simulink model "WholeSys0720_Simplified"  (Simulink 7.5)
settings: Solver=ode15s  StartTime=0.0  StopTime=10.0  MaxStep=0.2  RelTol=1e-3
undefined symbols (not defined in the file or in its folder): des_attributefunction_support, des_figposition, des_subsystemblock, des_subsysteminport, des_subsystemoutport, des_subsystemsupportblock, DiscIntNeverNeededParam, mm, Radius, sigbuilder_block, X, Y
libraries: simeventssink1 x10, simeventsattributes2 x5, simeventsgenerators1 x4, dspmathops x3, simeventstranslate1 x3, dspsigops x2, dspsrcs4 x2, simeventsgates1 x1, simeventsrouting1 x1, simeventsserver1 x1
settings Model: Creator=Administrator  LastModifiedBy=Administrator
settings DebuggingCC: StrictBusMsg=Warning
settings SimEventsCC: propDiagAttribOutput=1  propDiagFcnCallOutput=1  propDiagStatOutput=0

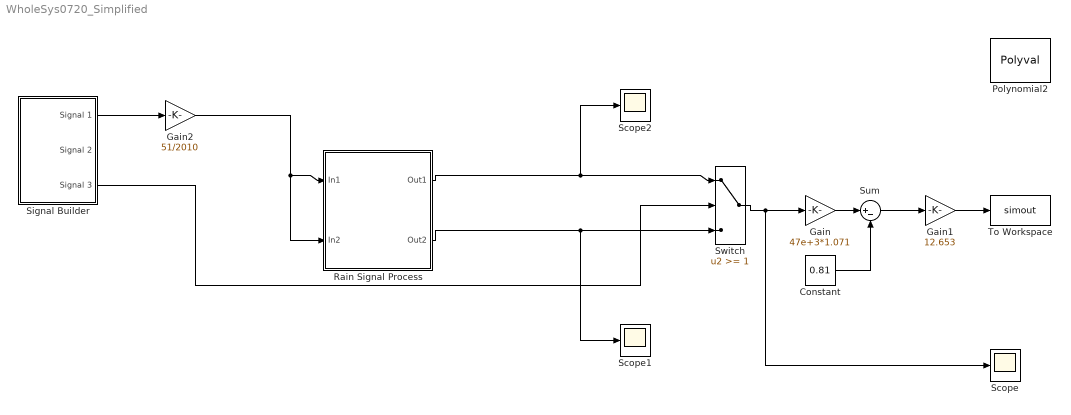
== system WholeSys0720_Simplified ==
  Constant : Constant  Value=0.81  OutDataType=sfix(16)  OutScaling=2^0
  Gain : Gain  Gain=47e+3*1.071  ParameterDataType=sfix(16)  ParameterScaling=2^0  OutDataType=sfix(16)  OutScaling=2^0
  Gain1 : Gain  Gain=12.653  ParameterDataType=sfix(16)  ParameterScaling=2^0  OutDataType=sfix(16)  OutScaling=2^0
  Gain2 : Gain  Gain=51/2010  ParameterDataType=fixdt(1, 16)  ParameterScaling=2^0  OutDataType=fixdt(1, 16)  OutScaling=2^0
  Polynomial2 : Polyval  Coefs=[ 1 ]
  Rain Signal Process : Subsystem
  Scope : Scope
      settings: YMin=-0.5  YMax=1.5  MaxDataPoints=100000
  Scope1 : Scope
      settings: YMin=-0.5  YMax=1  SaveName=ScopeData2  MaxDataPoints=100000
  Scope2 : Scope
      settings: YMin=-0.5  YMax=1  SaveName=ScopeData9  MaxDataPoints=100000
  Signal Builder : Subsystem  Tag=STV Subsys  LoadFcn=sigbuilder_block('load');  StartFcn=sigbuilder_block('start');  StopFcn=sigbuilder_block('stop');  ClipboardFcn=sigbuilder_block('clipboard');  mask(Sigbuilder block){}
      mask help: Create and generate interchangeable groups of signals whose waveforms are piecewise linear.
      mask init:
      | if ~strcmp(get_param(bdroot(gcbh),'SimulationStatus'),'stopped') tuvar = sigbuilder_block('maskInit'); end
      settings: CopyFcn=sigbuilder_block('copy');  DeleteFcn=sigbuilder_block('delete');  ModelCloseFcn=sigbuilder_block('modelClose');  PreSaveFcn=sigbuilder_block('preSave');  NameChangeFcn=sigbuilder_block('namechange');  OpenFcn=sigbuilder_block('open',[437.25 199.5 550.5 399.75 ]);  CloseFcn=sigbuilder_block('close');
      mask Display: plot(0,0,100,100,[10,10,40,40,10],[80,20,20,80,80],[40,10],[50,50], [40,27,10],[65,72,56],[40,25,25,10],[28,28,43,43]);
  Sum : Sum  Inputs=|+-  OutDataType=sfix(16)  OutScaling=2^0
  Switch : Switch  Threshold=1  OutDataType=fixdt(1, 16)  OutScaling=2^0
  To Workspace : ToWorkspace  VariableName=simout  SampleTime=-1  SaveFormat=Structure
  wires:
  Gain2/1 -> Rain Signal Process/1(In1), Rain Signal Process/2(In2)
  Gain/1 -> Sum/1
  Constant/1 -> Sum/2
  Sum/1 -> Gain1/1
  Gain1/1 -> To Workspace/1
  Rain Signal Process/1(Out1) -> Switch/1, Scope2/1
  Rain Signal Process/2(Out2) -> Switch/3, Scope1/1
  Switch/1 -> Gain/1, Scope/1
  Signal Builder/1(Signal 1) -> Gain2/1
  Signal Builder/3(Signal 3) -> Switch/2

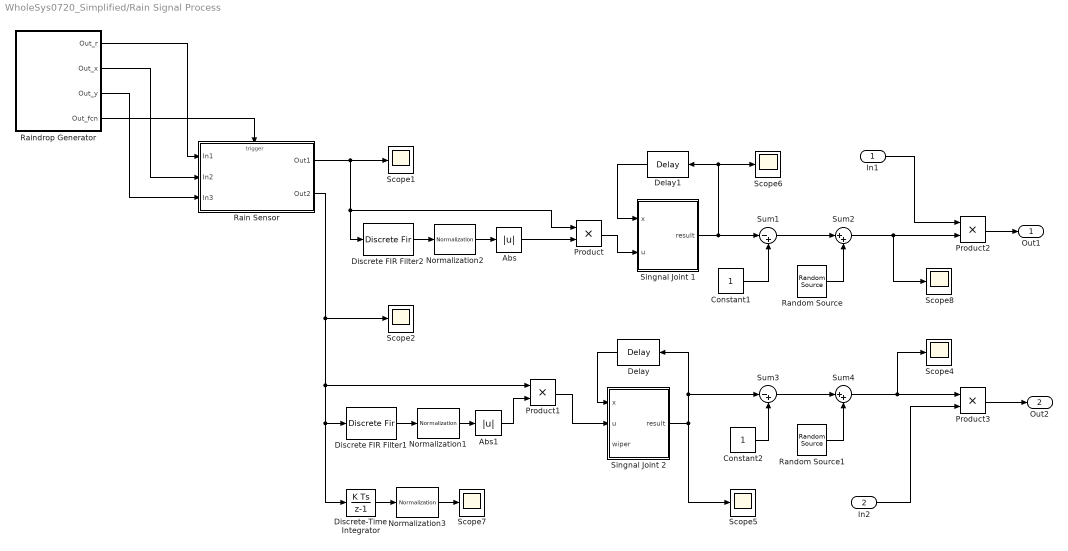
== system WholeSys0720_Simplified/Rain Signal Process ==
  In1 : Inport  OutDataType=sfix(16)  OutScaling=2^0
  In2 : Inport  Port=2  OutDataType=sfix(16)  OutScaling=2^0
  Abs : Abs  OutDataType=sfix(16)  OutScaling=2^0  OutDataTypeStr=Inherit: Inherit via internal rule
  Abs1 : Abs  OutDataType=sfix(16)  OutScaling=2^0
  Constant1 : Constant  OutDataType=sfix(16)  OutScaling=2^0
  Constant2 : Constant  OutDataType=sfix(16)  OutScaling=2^0
  Delay : dspsigops/Delay  dly_unit=Samples  delay=1  ic_detail=off  dif_ic_for_ch=off  dif_ic_for_dly=off  ic=0  reset_popup=None
  Delay1 : dspsigops/Delay  dly_unit=Samples  delay=1  ic_detail=off  dif_ic_for_ch=off  dif_ic_for_dly=off  ic=0  reset_popup=None
  Discrete FIR Filter1 : DiscreteFir  NumCoeffs=[1 0 0 -1]
  Discrete FIR Filter2 : DiscreteFir  NumCoeffs=[1 0 0 -1]
  Discrete-Time Integrator : DiscreteIntegrator  SampleTime=0.0001  OutDataType=fixdt(1, 16)  OutScaling=2^0  ICPrevOutput=DiscIntNeverNeededParam  ICPrevScaledInput=DiscIntNeverNeededParam
  Normalization1 : dspmathops/Normalization  DialogController=dspDDGCreate  DialogControllerArgs=DataTag0  NormType=2-norm  Bias=1e-10  NormOver=Each column  ColComp=on  Dimension=1  outputDataTypeStr=Inherit: Same as product output  outputLastDataTypeStr=Inherit: Same as product output  outputMin=[]  outputMax=[]  accumDataTypeStr=Inherit: Same as product output  accumLastDataTypeStr=Inherit: Same as product output  roundingMode=Floor  overflowMode=off
  Normalization2 : dspmathops/Normalization  DialogController=dspDDGCreate  DialogControllerArgs=DataTag1  NormType=2-norm  Bias=1e-10  NormOver=Each column  ColComp=on  Dimension=1  outputDataTypeStr=Inherit: Same as product output  outputLastDataTypeStr=Inherit: Same as product output  outputMin=[]  outputMax=[]  accumDataTypeStr=Inherit: Same as product output  accumLastDataTypeStr=Inherit: Same as product output  roundingMode=Floor  overflowMode=off
  Normalization3 : dspmathops/Normalization  DialogController=dspDDGCreate  DialogControllerArgs=DataTag2  NormType=2-norm  Bias=1e-10  NormOver=Each column  ColComp=on  Dimension=1  outputDataTypeStr=Inherit: Same as product output  outputLastDataTypeStr=Inherit: Same as product output  outputMin=[]  outputMax=[]  accumDataTypeStr=Inherit: Same as product output  accumLastDataTypeStr=Inherit: Same as product output  roundingMode=Floor  overflowMode=off
  Product : Product  OutDataType=sfix(16)  OutScaling=2^0  SampleTime=0.0001  RndMeth=Zero
  Product1 : Product  OutDataType=sfix(16)  OutScaling=2^0  SampleTime=0.0001  RndMeth=Zero
  Product2 : Product  OutDataType=fixdt(1, 16)  OutScaling=2^0  SampleTime=0.0001  RndMeth=Zero
  Product3 : Product  OutDataType=fixdt(1, 16)  OutScaling=2^0  SampleTime=0.0001  RndMeth=Zero
  Rain Sensor : Subsystem  TreatAsAtomicUnit=on
  Raindrop Generator : Subsystem
  Random Source : dspsrcs4/Random Source  SrcType=Gaussian  NormMethod=Ziggurat  CltLength=12  MinVal=0  MaxVal=1  MeanVal=0  VarVal=0.00001  RepMode=Not repeatable  rawSeed=1  IsInherit=off  SampMode=Discrete  SampTime=0.001  SampFrame=1  DataType=Double  OutComplex=Real
  Random Source1 : dspsrcs4/Random Source  SrcType=Gaussian  NormMethod=Ziggurat  CltLength=12  MinVal=0  MaxVal=1  MeanVal=0  VarVal=0.00001  RepMode=Not repeatable  rawSeed=1  IsInherit=off  SampMode=Discrete  SampTime=0.001  SampFrame=1  DataType=Double  OutComplex=Real
  Scope{1..2,4..8} (7 alike) : Scope
      Scope1 settings: MaxDataPoints=150000
      Scope2 settings: SaveName=ScopeData4  MaxDataPoints=150000
      Scope4 settings: SaveName=ScopeData3  MaxDataPoints=150000
      Scope5 settings: TimeRange=10  YMin=-0.1  YMax=1.5  SaveName=ScopeData5  MaxDataPoints=150000
      Scope6 settings: TimeRange=10  YMin=-0.1  YMax=1.5  SaveName=ScopeData6  MaxDataPoints=150000
      Scope7 settings: TimeRange=10  YMin=-0.1  YMax=1.5  SaveName=ScopeData7  MaxDataPoints=150000
      Scope8 settings: SaveName=ScopeData8  MaxDataPoints=150000
  Singnal Joint 1 : Stateflow chart  TreatAsAtomicUnit=on
  Singnal Joint 2 : Stateflow chart  TreatAsAtomicUnit=on
  Sum1 : Sum  Inputs=|-+  OutDataType=sfix(16)  OutScaling=2^0
  Sum2 : Sum  Inputs=|++  OutDataType=sfix(16)  OutScaling=2^0
  Sum3 : Sum  Inputs=|-+  OutDataType=sfix(16)  OutScaling=2^0
  Sum4 : Sum  Inputs=|++  OutDataType=sfix(16)  OutScaling=2^0
  Out1 : Outport  OutDataType=sfix(16)  OutScaling=2^0
  Out2 : Outport  Port=2  OutDataType=sfix(16)  OutScaling=2^0
  wires:
  Raindrop Generator/1(Out_r) -> Rain Sensor/1(In1)
  Raindrop Generator/2(Out_x) -> Rain Sensor/2(In2)
  Raindrop Generator/3(Out_y) -> Rain Sensor/3(In3)
  Raindrop Generator/4(Out_fcn) -> Rain Sensor/Trigger
  Rain Sensor/2(Out2) -> Product1/1, Discrete FIR Filter1/1, Discrete-Time Integrator/1, Scope2/1
  Rain Sensor/1(Out1) -> Discrete FIR Filter2/1, Product/1, Scope1/1
  Discrete FIR Filter1/1 -> Normalization1/1
  Normalization1/1 -> Abs1/1
  Abs/1 -> Product/2
  Abs1/1 -> Product1/2
  Normalization2/1 -> Abs/1
  Discrete FIR Filter2/1 -> Normalization2/1
  Product1/1 -> Singnal Joint 2/2(u)
  Product/1 -> Singnal Joint 1/2(u)
  Singnal Joint 1/1(result) -> Sum1/1, Delay1/1, Scope6/1
  Constant1/1 -> Sum1/2
  Sum1/1 -> Sum2/1
  Random Source/1 -> Sum2/2
  Constant2/1 -> Sum3/2
  Sum3/1 -> Sum4/1
  Random Source1/1 -> Sum4/2
  Singnal Joint 2/1(result) -> Sum3/1, Delay/1, Scope5/1
  Delay/1 -> Singnal Joint 2/1(x)
  Delay1/1 -> Singnal Joint 1/1(x)
  Discrete-Time Integrator/1 -> Normalization3/1
  Normalization3/1 -> Scope7/1
  Sum4/1 -> Product3/1, Scope4/1
  In2/1 -> Product3/2
  Sum2/1 -> Product2/2, Scope8/1
  Product3/1 -> Out2/1
  Product2/1 -> Out1/1
  In1/1 -> Product2/1

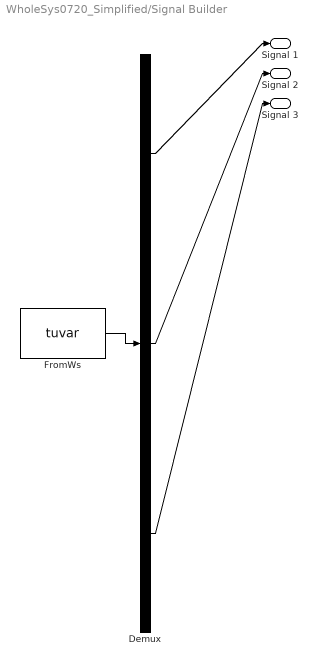
== system WholeSys0720_Simplified/Signal Builder ==
  Demux : Demux  Tag=STV Demux  Outputs=3
  FromWs : FromWorkspace  Tag=STV FromWs  VariableName=tuvar  SampleTime=0  SigBuilderData=DataTag33  VnvData=DataTag34
      SigBuilderData=|
      | common.afterFinalStr = 'Extrapolate'
      | common.sampleTime = 0
      | dataSet.timeRange = [0 10]
      | dataSet.name = 'Group 1'
      | sbobj.Groups.Name = 'Group 1'
      | sbobj.Groups.Signals(1).Name = 'Signal 1'
      | sbobj.Groups.Signals(1).XData = [0 6e-05 6e-05 0.0025 0.0025 0.00256 0.00256 0.005 0.005 0.00506 0.00506 0.0075 ... (15988 elements, 1x15988)]
      | sbobj.Groups.Signals(1).YData = [6 6 0 0 6 6 0 0 6 6 0 0 ... (15988 elements, 1x15988)]
      | sbobj.Groups.Signals(2).Name = 'Signal 2'
      | sbobj.Groups.Signals(2).XData = [0 0.0025 0.0025 0.005 0.005 0.0075 0.0075 0.01 0.01 0.0125 0.0125 0.015 ... (8000 elements, 1x8000)]
      | sbobj.Groups.Signals(2).YData = [2 2 0 0 2 2 0 0 2 2 0 0 ... (8000 elements, 1x8000)]
      | sbobj.Groups.Signals(3).Name = 'Signal 3'
      | sbobj.Groups.Signals(3).XData = [0 0.0025 0.0025 0.005 0.005 0.0075 0.0075 0.01 0.01 0.0125 0.0125 0.015 ... (8000 elements, 1x8000)]
      | sbobj.Groups.Signals(3).YData = [4 4 0 0 4 4 0 0 4 4 0 0 ... (8000 elements, 1x8000)]
  Signal 1 : Outport  Tag=STV Outport
  Signal 2 : Outport  Tag=STV Outport  Port=2
  Signal 3 : Outport  Tag=STV Outport  Port=3
  wires:
  FromWs/1 -> Demux/1
  Demux/1 -> Signal 1/1
  Demux/2 -> Signal 2/1
  Demux/3 -> Signal 3/1

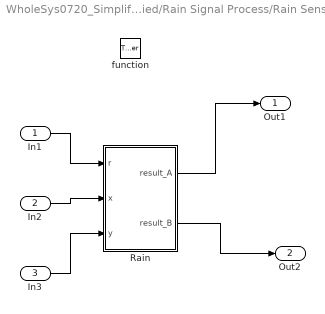
== system WholeSys0720_Simplified/Rain Signal Process/Rain Sensor ==
  In1 : Inport  OutDataType=sfix(16)  OutScaling=2^0
  In2 : Inport  Port=2  OutDataType=sfix(16)  OutScaling=2^0
  In3 : Inport  Port=3  OutDataType=sfix(16)  OutScaling=2^0
  function : TriggerPort  TriggerType=function-call
  Rain : Stateflow chart  TreatAsAtomicUnit=on
  Out1 : Outport  OutDataType=sfix(16)  OutScaling=2^0
  Out2 : Outport  Port=2  OutDataType=sfix(16)  OutScaling=2^0
  wires:
  In1/1 -> Rain/1(r)
  In2/1 -> Rain/2(x)
  In3/1 -> Rain/3(y)
  Rain/1(result_A) -> Out1/1
  Rain/2(result_B) -> Out2/1

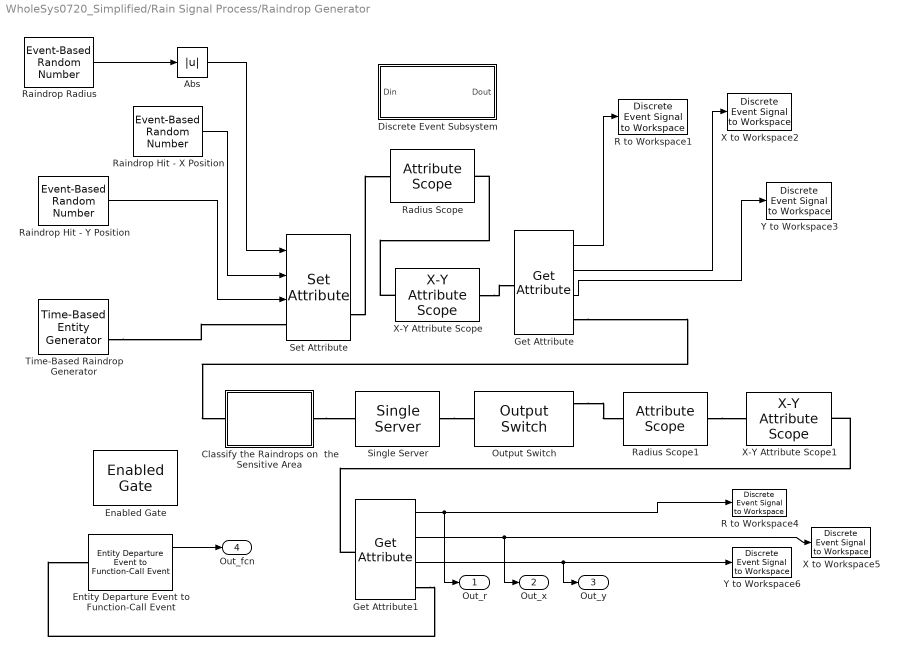
== system WholeSys0720_Simplified/Rain Signal Process/Raindrop Generator ==
  Abs : Abs  OutDataType=sfix(16)  OutScaling=2^0
  Classify the Raindrops on  the Sensitive Area : Subsystem  LoadFcn=des_attributefunction_support(gcb,'LoadFcn');  StartFcn=des_attributefunction_support(gcb,'StartFcn');  mask(Attribute Function){OutputNamePrefix=out_}
      mask prompts: OutputNamePrefix "Prefix name"
      settings: CopyFcn=des_attributefunction_support(gcb,'CopyFcn');  OpenFcn=des_attributefunction_support(gcb,'OpenFcn');  ErrorFcn=des_error_redirect
      mask Help: helpview(simeventsbhelp('attributefunction'))
      mask Display: image(des_iconLoad('attribFunction.jpg'),'center');
  Discrete Event Subsystem : Subsystem  LoadFcn=des_subsystemblock(gcb, 'load');  InitFcn=des_subsystemblock(gcb, 'init');  StartFcn=des_subsystemblock(gcb, 'start');  StopFcn=des_subsystemblock(gcb, 'stop');
      settings: CopyFcn=des_subsystemblock(gcb, 'copy');  DeleteFcn=des_subsystemblock(gcb, 'delete');  UndoDeleteFcn=des_subsystemblock(gcb, 'undodelete');  ModelCloseFcn=des_subsystemblock(gcb, 'modelclose');  PreSaveFcn=des_subsystemblock(gcb, 'presave');  NameChangeFcn=des_subsystemblock(gcb, 'namechange');  OpenFcn=des_subsystemblock(gcb, 'open');  ParentCloseFcn=des_subsystemblock(gcb, 'parentclose');  ErrorFcn=des_subsystemerror
      mask Type: Discrete Event Subsystem
      mask Help: helpview(simeventsbhelp);
  Enabled Gate : simeventsgates1/Enabled Gate  Priority=1  SystemSampleTime=-1  SpecifyEventPriority=off  PriorityGateEnableOpenClose=2000  StatNumberDeparted=Off
  Entity Departure Event to Function-Call Event : simeventstranslate1/Entity Departure Event to Function-Call Event  Priority=1  SystemSampleTime=-1  TimingFunctionCallF1=After entity departure  EnableE1Port=off  EnableF2Port=off  TimingFunctionCallF2=Before entity departure  EnableE2Port=off  StatNumberDeparted=Off  StatNumberF1Calls=Off  StatNumberF2Calls=Off  IsInsideAFB=off
  Get Attribute : simeventsattributes2/Get Attribute  Priority=1  DialogController=des_ddg_create  DialogControllerArgs=DataTag18  SystemSampleTime=-1  AttributeName=R|X|Y  AttributeMissing=Error|Error|Error  AttributeDefaultValue=1|1|1  AttributeSendTiming=After entity departure|After entity departure|After entity departure  AttributeTreatAsVector=1|1|1  StatNumberDeparted=Off  EvaluatedDefaultAttributeValue={[];[];[]}
  Get Attribute1 : simeventsattributes2/Get Attribute  Priority=1  DialogController=des_ddg_create  DialogControllerArgs=DataTag20  SystemSampleTime=-1  AttributeName=R|X|Y  AttributeMissing=Error|Error|Error  AttributeDefaultValue=1|1|1  AttributeSendTiming=After entity departure|After entity departure|After entity departure  AttributeTreatAsVector=1|1|1  StatNumberDeparted=Off  EvaluatedDefaultAttributeValue={[];[];[]}
  Output Switch : simeventsrouting1/Output Switch  Priority=1  SystemSampleTime=-1  NumberOutputPorts=2  SwitchingCriterion=From attribute  InitialSeed=34567  AttributeName=Flag  InitialConditionsOpt=off  InitialConditions=1  EntityBufferOpt=off  SpecifyEventPriority=off  PriorityOutputSwitchSelectPort=4100  TimeoutPortOpt=off  StatNumberDeparted=Off  StatNumberTimedOut=Off  StatPendingEntity=Off  StatLastDeparturePort=Off  EvaluatedNumPorts=2
  R to Workspace1 : simeventssink1/Discrete Event Signal to Workspace  SystemSampleTime=-1  VariableName=DataR_WS  SaveFormat=Structure With Time  IsMonitorOnly=off  IsRecordIC=off
  R to Workspace4 : simeventssink1/Discrete Event Signal to Workspace  SystemSampleTime=-1  VariableName=DataR  SaveFormat=Structure With Time  IsMonitorOnly=off  IsRecordIC=off
  Radius Scope : simeventssink1/Attribute Scope  Priority=1  SystemSampleTime=-1  PlotType=Stem  InputType=Attribute  NumInputs=1  AttributeNameY=R  XInputOptionSignal=Event time  XInputOptionEntity=Event time  AttributeNameX=Count  EnableEntityOutport=on  XMin=0  XMax=10  XLimitExceededOption=Stretch axis limits  YLimitExceededOption=Keep axis limits unchanged  AxisGrid=on  AxisLegend=off  LineDisables=""  LineColors="1  0  0"  LineStyles=-  LineMarkers=.  OpenScopeAtSimStart=on  Title=Size/Time of Raindrop Arrival  YLabel=Radius/mm  XLabel=Time/sec  FigurePosition=des_figposition([5 25 25 25])  AxisZoom=off  DataStoreOption=Limited  DataPointsLimit=50000  StatNumberArrived=Off  ShowCountPlotted=off  ShowToolbar=on
      settings: YMin=-1  YMax=5
  Radius Scope1 : simeventssink1/Attribute Scope  Priority=1  SystemSampleTime=-1  PlotType=Stem  InputType=Attribute  NumInputs=1  AttributeNameY=R  XInputOptionSignal=Event time  XInputOptionEntity=Event time  AttributeNameX=Count  EnableEntityOutport=on  XMin=0  XMax=10  XLimitExceededOption=Stretch axis limits  YLimitExceededOption=Keep axis limits unchanged  AxisGrid=on  AxisLegend=off  LineDisables=""  LineColors="1  0  0"  LineStyles=-  LineMarkers=.  OpenScopeAtSimStart=on  Title=Size/Time of Raindrop Arrival  YLabel=Radius/mm  XLabel=Time/sec  FigurePosition=des_figposition([5 25 25 25])  AxisZoom=off  DataStoreOption=Limited  DataPointsLimit=10000  StatNumberArrived=Off  ShowCountPlotted=on  ShowToolbar=on
      settings: YMin=-1  YMax=5
  Raindrop Hit - X Position : simeventsgenerators1/Signal Generators/Event-Based Random Number  SystemSampleTime=-1  distribution=Uniform  meanExp=1  minUnif=-750  maxUnif=750  pOneBern=0.25  pSuccessBino=0.5  numTrialBino=1  meanNorm=0  stdNorm=1  minTri=1  maxTri=3  modeTri=2  thresholdLogn=0  scaleLogn=1  shapeLogn=1  pSuccessGeo=0.5  meanPoiss=1  thresholdLogl=0  scaleLogl=1  thresholdGam=0  scaleGam=1  shapeGam=1  minBeta=0  maxBeta=1  shape1Beta=1  shape2Beta=1  minUnid=0  maxUnid=1  numValueUnid=2  thresholdWbl=0  scaleWbl=1  shapeWbl=1  valueVecCont=[0 1]  cdfVecCont=[0 1]  valueVecDisc=[0 1]  probVecDisc=[0.5 0.5]  seed=25  IsProcessed=on  isConnected=1
  Raindrop Hit - Y Position : simeventsgenerators1/Signal Generators/Event-Based Random Number  SystemSampleTime=-1  distribution=Uniform  meanExp=1  minUnif=-910  maxUnif=90  pOneBern=0.25  pSuccessBino=0.5  numTrialBino=1  meanNorm=0  stdNorm=1  minTri=1  maxTri=3  modeTri=2  thresholdLogn=0  scaleLogn=1  shapeLogn=1  pSuccessGeo=0.5  meanPoiss=1  thresholdLogl=0  scaleLogl=1  thresholdGam=0  scaleGam=1  shapeGam=1  minBeta=0  maxBeta=1  shape1Beta=1  shape2Beta=1  minUnid=0  maxUnid=1  numValueUnid=2  thresholdWbl=0  scaleWbl=1  shapeWbl=1  valueVecCont=[0 1]  cdfVecCont=[0 1]  valueVecDisc=[0 1]  probVecDisc=[0.5 0.5]  seed=111  IsProcessed=on  isConnected=1
  Raindrop Radius : simeventsgenerators1/Signal Generators/Event-Based Random Number  SystemSampleTime=-1  distribution=Gaussian (normal)  meanExp=1  minUnif=1  maxUnif=1  pOneBern=0.25  pSuccessBino=0.5  numTrialBino=1  meanNorm=1.5  stdNorm=.5  minTri=1  maxTri=3  modeTri=2  thresholdLogn=0  scaleLogn=1  shapeLogn=1  pSuccessGeo=0.5  meanPoiss=1  thresholdLogl=0  scaleLogl=1  thresholdGam=0  scaleGam=1  shapeGam=1  minBeta=0  maxBeta=1  shape1Beta=1  shape2Beta=1  minUnid=0  maxUnid=1  numValueUnid=2  thresholdWbl=0  scaleWbl=1  shapeWbl=1  valueVecCont=[0 1]  cdfVecCont=[0 1]  valueVecDisc=[0 1]  probVecDisc=[0.5 0.5]  seed=11  IsProcessed=on  isConnected=1
  Set Attribute : simeventsattributes2/Set Attribute  Priority=1  DialogController=des_ddg_create  DialogControllerArgs=DataTag25  SystemSampleTime=-1  AttributeFrom=Signal port|Signal port|Signal port  AttributeName=R|X|Y  AttributeTreatAsVector=1|1|1  AttributeValue=1|1|1  AttributeCreate=on  StatNumberDeparted=On  EvaluatedAttributeValue={[];[];[]}
  Single Server : simeventsserver1/Single Server  Priority=1  SystemSampleTime=-1  ServiceTimeFrom=Dialog  ServiceTime=0  AttributeName=ServiceTime  PriorityServiceCompletion=500  PermitPreemption=off  SortingAttributeName=PriorityAttributeName  SortingDirection=Ascending  WriteToAttribute=off  ResidualAttributeName=ResidualServiceTime  CreateAttribute=on  EnableTOPort=off  StatNumberDeparted=Off  StatNumberInBlock=Off  StatNumberPreempted=Off  StatPendingEntity=Off  StatAverageWait=Off  StatUtilization=Off  StatNumberTimedout=Off
  Time-Based Raindrop Generator : simeventsgenerators1/Entity Generators/Time-Based Entity Generator  Priority=1  DialogController=des_ddg_create  DialogControllerArgs=DataTag28  SystemSampleTime=-1  GenerateEntitiesUpon=Intergeneration time from dialog  Distribution=Exponential  Minimum=0  Maximum=1  Mean=2e-4  InitialSeed=12345  Period=1  PriorityEntityGeneration=300  GenerateEntityAtSimulationStart=on  ResponseWhenBlocked=Pause generation  ResponseWhenUnblocked=Immediate restart  EntityType=Standard  StatNumberDeparted=On  StatPendingEntity=Off  StatAverageIntergenerationTime=Off
  X to Workspace2 : simeventssink1/Discrete Event Signal to Workspace  SystemSampleTime=-1  VariableName=DataX_WS  SaveFormat=Structure With Time  IsMonitorOnly=off  IsRecordIC=off
  X to Workspace5 : simeventssink1/Discrete Event Signal to Workspace  SystemSampleTime=-1  VariableName=DataX  SaveFormat=Structure With Time  IsMonitorOnly=off  IsRecordIC=off
  X-Y Attribute Scope : simeventssink1/X-Y Attribute Scope  Priority=1  SystemSampleTime=-1  PlotType=Stair  InputType=Attribute  NumInputs=1  AttributeNameY=Y  XInputOptionSignal=Event time  XInputOptionEntity=Attribute  AttributeNameX=X  EnableEntityOutport=on  XMin=-800  XMax=800  XLimitExceededOption=Keep axis limits unchanged  YLimitExceededOption=Keep axis limits unchanged  AxisGrid=on  AxisLegend=off  LineDisables=""  LineColors=b  LineStyles=None  LineMarkers=.  OpenScopeAtSimStart=on  Title=Position of Raindrop Hits  YLabel=Y/mm  XLabel=X/mm  FigurePosition=des_figposition([5 25 25 25])  AxisZoom=off  DataStoreOption=Limited  DataPointsLimit=10000  StatNumberArrived=Off  ShowCountPlotted=on  ShowToolbar=on
      settings: YMin=-990  YMax=170
  X-Y Attribute Scope1 : simeventssink1/X-Y Attribute Scope  Priority=1  SystemSampleTime=-1  PlotType=Stair  InputType=Attribute  NumInputs=1  AttributeNameY=Y  XInputOptionSignal=Event time  XInputOptionEntity=Attribute  AttributeNameX=X  EnableEntityOutport=on  XMin=-12.5  XMax=12.5  XLimitExceededOption=Keep axis limits unchanged  YLimitExceededOption=Keep axis limits unchanged  AxisGrid=on  AxisLegend=off  LineDisables=""  LineColors=b  LineStyles=None  LineMarkers=diamond  OpenScopeAtSimStart=on  Title=Position of Raindrop Hits  YLabel=Y/mm  XLabel=X/mm  FigurePosition=des_figposition([5 25 25 25])  AxisZoom=off  DataStoreOption=Limited  DataPointsLimit=10000  StatNumberArrived=Off  ShowCountPlotted=on  ShowToolbar=on
      settings: YMin=-12.5  YMax=12.5
  Y to Workspace3 : simeventssink1/Discrete Event Signal to Workspace  SystemSampleTime=-1  VariableName=DataY_WS  SaveFormat=Structure With Time  IsMonitorOnly=off  IsRecordIC=off
  Y to Workspace6 : simeventssink1/Discrete Event Signal to Workspace  SystemSampleTime=-1  VariableName=DataY  SaveFormat=Structure With Time  IsMonitorOnly=off  IsRecordIC=off
  Out_r : Outport  OutDataType=sfix(16)  OutScaling=2^0
  Out_x : Outport  Port=2  OutDataType=sfix(16)  OutScaling=2^0
  Out_y : Outport  Port=3  OutDataType=sfix(16)  OutScaling=2^0
  Out_fcn : Outport  Port=4  OutDataType=sfix(16)  OutScaling=2^0
  wires:
  Raindrop Hit - X Position/1 -> Set Attribute/2
  Raindrop Hit - Y Position/1 -> Set Attribute/3
  Get Attribute/1 -> R to Workspace1/1
  Get Attribute/2 -> X to Workspace2/1
  Get Attribute/3 -> Y to Workspace3/1
  Raindrop Radius/1 -> Abs/1
  Abs/1 -> Set Attribute/1
  Get Attribute1/1 -> Out_r/1, R to Workspace4/1
  Get Attribute1/2 -> X to Workspace5/1, Out_x/1
  Get Attribute1/3 -> Y to Workspace6/1, Out_y/1
  Entity Departure Event to Function-Call Event/1 -> Out_fcn/1
  connections:
  Get Attribute/RConn1 -- Classify the Raindrops on  the Sensitive Area/LConn1
  Set Attribute/RConn1 -- Radius Scope/LConn1
  X-Y Attribute Scope/LConn1 -- Radius Scope/RConn1
  Get Attribute1/LConn1 -- X-Y Attribute Scope1/RConn1
  Single Server/RConn1 -- Output Switch/LConn1
  Radius Scope1/RConn1 -- X-Y Attribute Scope1/LConn1
  Classify the Raindrops on  the Sensitive Area/RConn1 -- Single Server/LConn1
  Output Switch/RConn1 -- Radius Scope1/LConn1
  Time-Based Raindrop Generator/RConn1 -- Set Attribute/LConn1
  X-Y Attribute Scope/RConn1 -- Get Attribute/LConn1
  Get Attribute1/RConn1 -- Entity Departure Event to Function-Call Event/LConn1

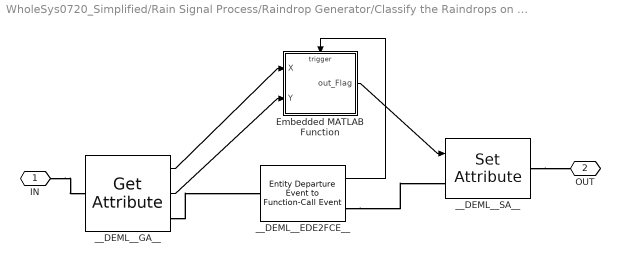
== system WholeSys0720_Simplified/Rain Signal Process/Raindrop Generator/Classify the Raindrops on  the Sensitive Area ==
  Embedded MATLAB Function : Stateflow chart  TreatAsAtomicUnit=on
      settings: PropExecContextOutsideSubsystem=on
  __DEML__EDE2FCE__ : simeventstranslate1/Entity Departure Event to Function-Call Event  Priority=1  SystemSampleTime=-1  TimingFunctionCallF1=Before entity departure  EnableE1Port=off  EnableF2Port=off  TimingFunctionCallF2=Before entity departure  EnableE2Port=off  StatNumberDeparted=Off  StatNumberF1Calls=Off  StatNumberF2Calls=Off  IsInsideAFB=on
  __DEML__GA__ : simeventsattributes2/Get Attribute  Priority=1  DialogController=des_ddg_create  DialogControllerArgs=DataTag5  SystemSampleTime=-1  AttributeName=X|Y  AttributeMissing=Error|Error  AttributeDefaultValue=1|1  AttributeSendTiming=Before entity departure|Before entity departure  AttributeTreatAsVector=1|1  StatNumberDeparted=Off  EvaluatedDefaultAttributeValue={[];[]}
  __DEML__SA__ : simeventsattributes2/Set Attribute  Priority=1  DialogController=des_ddg_create  DialogControllerArgs=DataTag7  SystemSampleTime=-1  AttributeFrom=Signal port  AttributeName=Flag  AttributeTreatAsVector=1  AttributeValue=1  AttributeCreate=on  StatNumberDeparted=Off  EvaluatedAttributeValue={[]}
  IN : PMIOPort  Port=1  Side=Left
  OUT : PMIOPort  Port=2  Side=Right
  wires:
  __DEML__EDE2FCE__/1 -> Embedded MATLAB Function/Trigger
  __DEML__GA__/1 -> Embedded MATLAB Function/1(X)
  __DEML__GA__/2 -> Embedded MATLAB Function/2(Y)
  Embedded MATLAB Function/1(out_Flag) -> __DEML__SA__/1
  connections:
  __DEML__SA__/RConn1 -- OUT/RConn1
  IN/RConn1 -- __DEML__GA__/LConn1
  __DEML__GA__/RConn1 -- __DEML__EDE2FCE__/LConn1
  __DEML__EDE2FCE__/RConn1 -- __DEML__SA__/LConn1

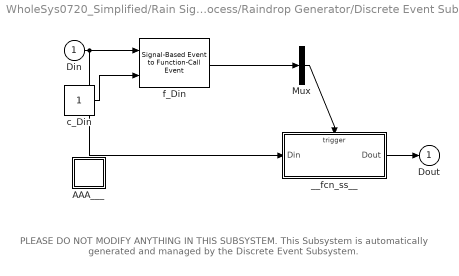
== system WholeSys0720_Simplified/Rain Signal Process/Raindrop Generator/Discrete Event Subsystem ==
  note: PLEASE DO NOT MODIFY ANYTHING IN THIS SUBSYSTEM.
      | This Subsystem is automatically generated and
      | managed by the Discrete Event Subsystem.
  Din : Inport  DataType=double  OutDataType=sfix(16)  OutScaling=2^0  OutDataTypeStr=double
  AAA___ : Subsystem  LoadFcn=des_subsystemsupportblock(gcb, 'load');  InitFcn=des_subsystemsupportblock(gcb, 'init');  StartFcn=des_subsystemsupportblock(gcb, 'start');  StopFcn=des_subsystemsupportblock(gcb, 'stop');
      settings: CopyFcn=des_subsystemsupportblock(gcb, 'copy');  DeleteFcn=des_subsystemsupportblock(gcb, 'delete');  UndoDeleteFcn=des_subsystemsupportblock(gcb, 'undodelete');  ModelCloseFcn=des_subsystemsupportblock(gcb, 'modelclose');  PreSaveFcn=des_subsystemsupportblock(gcb, 'presave');  NameChangeFcn=des_subsystemsupportblock(gcb, 'namechange');  OpenFcn=des_subsystemsupportblock(gcb, 'open');  ParentCloseFcn=des_subsystemsupportblock(gcb, 'parentclose');
  Mux : Mux  Inputs=1
  __fcn_ss__ : Subsystem  TreatAsAtomicUnit=on
      settings: PropExecContextOutsideSubsystem=on
  c_Din : Constant  OutDataType=sfix(16)  OutScaling=2^0
  f_Din : simeventstranslate1/Signal-Based Event to Function-Call Event  Priority=1  SystemSampleTime=-1  GenerateFunctionCallUpon=Sample time hit from port ts  SignalEdgeOption=Rising  EnableE1Port=on  EnableF2Port=off  EnableE2Port=off  SpecifyEventPriority=off  PriorityFunctionCall=20  FunctionCallDelayFrom=Dialog  DelayFunctionCall=0  StatNumberF1Calls=Off  StatNumberF2Calls=Off  MaskBlockType=DESS_EVENT_PORT
  Dout : Outport  OutDataType=sfix(16)  OutScaling=2^0
  wires:
  __fcn_ss__/1(Dout) -> Dout/1
  f_Din/1 -> Mux/1
  c_Din/1 -> f_Din/2
  Mux/1 -> __fcn_ss__/Trigger
  Din/1 -> f_Din/1, __fcn_ss__/1(Din)

== system WholeSys0720_Simplified/Rain Signal Process/Raindrop Generator/Discrete Event Subsystem/AAA___ ==

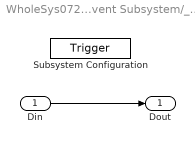
== system WholeSys0720_Simplified/Rain Signal Process/Raindrop Generator/Discrete Event Subsystem/__fcn_ss__ ==
  Din : Inport  LoadFcn=des_subsysteminport(gcb, 'load');  InitFcn=des_subsysteminport(gcb, 'init');  StartFcn=des_subsysteminport(gcb, 'start');  StopFcn=des_subsysteminport(gcb, 'stop');  OutDataType=sfix(16)  OutScaling=2^0  mask(Discrete Event Inport){PermitSubsystemEvents=on, TypeOfEvent=Sample time hit, SignalEdgeOption=Rising, SpecifyEventPriority=off, PrioritySubsystemEvent=20}
      mask prompts: PermitSubsystemEvents "Execute subsystem upon signal-based events"; TypeOfEvent "Type of signal-based event:"; SignalEdgeOption "Type of change in signal value:"; SpecifyEventPriority "Resolve simultaneous signal updates according to event priority"; PrioritySubsystemEvent "Event priority:"
      mask help: Input port for a Discrete Event Subsystem block. This block can conditionally execute the subsystem upon signal-based events that meet specified criteria.
      mask init:
      | des_subsystemmask(gcb, 'init','apply')
      settings: CopyFcn=des_subsysteminport(gcb, 'copy');  DeleteFcn=des_subsysteminport(gcb, 'delete');  UndoDeleteFcn=des_subsysteminport(gcb, 'undodelete');  ModelCloseFcn=des_subsysteminport(gcb, 'modelclose');  PreSaveFcn=des_subsysteminport(gcb, 'presave');  NameChangeFcn=des_subsysteminport(gcb, 'namechange');  ParentCloseFcn=des_subsysteminport(gcb, 'parentclose');
      mask Help: helpview(simeventsbhelp);
      mask StyleString: checkbox,popup(Change in signal|Trigger|Sample time hit),popup(Rising|Falling|Either),checkbox,edit
      mask CallbackString: des_subsystemmask(gcb, 'cbPermitSubsystemEvents', 'noapply');|des_subsystemmask(gcb,'cbTypeOfEvent','noapply');||des_subsystemmask(gcb, 'cbSpecifyEventPriority', 'noapply');|
  Subsystem Configuration : TriggerPort  TriggerType=function-call
      settings: CopyFcn=des_subsystemconfigblock(gcb, 'copy');  DeleteFcn=des_subsystemconfigblock(gcb, 'delete');  UndoDeleteFcn=des_subsystemconfigblock(gcb, 'undodelete');
      mask Type: Subsystem Configuration
      mask Description: Configuration for a Discrete Event Subsystem block. Every discrete event subsystem window must contain exactly one copy of this configuration block. Do not delete this block.
      mask Help: helpview(simeventsbhelp);
      mask Display: disp('Do Not Delete');
  Dout : Outport  LoadFcn=des_subsystemoutport(gcb, 'load');  InitFcn=des_subsystemoutport(gcb, 'init');  StartFcn=des_subsystemoutport(gcb, 'start');  StopFcn=des_subsystemoutport(gcb, 'stop');  OutDataType=sfix(16)  OutScaling=2^0
      settings: CopyFcn=des_subsystemoutport(gcb, 'copy');  DeleteFcn=des_subsystemoutport(gcb, 'delete');  UndoDeleteFcn=des_subsystemoutport(gcb, 'undodelete');  ModelCloseFcn=des_subsystemoutport(gcb, 'modelclose');  PreSaveFcn=des_subsystemoutport(gcb, 'presave');  NameChangeFcn=des_subsystemoutport(gcb, 'namechange');  ParentCloseFcn=des_subsystemoutport(gcb, 'parentclose');
      mask Type: Discrete Event Outport
      mask Description: Provide an output port for a Discrete Event Subsystem block.
      mask Help: helpview(simeventsbhelp);
  wires:
  Din/1 -> Dout/1

== matlab function Rain Signal Process/Singnal Joint 2 ==
  data: x input double; u input double; result output double; wiper input double
function result = fcn(x, u, wiper)
% This block supports the Embedded MATLAB subset. 
% See the help menu for details. 

result=x*0.999+u;

== matlab function Rain Signal Process/Rain Sensor/Rain ==
  data: r input double; x input double; y input double; result_A output double; result_B output double
function [result_A, result_B]= fcn(r, x, y)
% This block supports the Embedded MATLAB subset. 
% See the help menu for details. 

eml.extrinsic('RaindropEffect_2Ch','RaindropEffect_A','RaindropEffect_B');
sig=double(zeros(2,1));
[sig(1),sig(2)]=RaindropEffect_2Ch(r,x,y);
result_A=sig(1);
result_B=sig(2);

== matlab function Rain Signal Process/Raindrop Generator/Classify the Raindrops on the Sensitive Area/Embedded MATLAB Function ==
  data: X input double; out_Flag output double; Y input double
  events: trigger input FUNCTION_CALL_EVENT
function out_Flag = fcn(X, Y)
%FCN    Access and modify attributes with Embedded MATLAB Function 
% 
% Input arguments must match the attribute names.
% Output arguments must be out_<AttributeName>,
% e.g., out_ServiceTime where ServiceTime is the attribute name.
% 
% The output attribute will be created if it is not present.
%

if abs(X)<12.5 && abs(Y)<12.50
    out_Flag=1;
else
    out_Flag=2;
end

== matlab function Rain Signal Process/Singnal Joint 1 ==
  data: x input double; u input double; result output double
function result = fcn(x, u)
% This block supports the Embedded MATLAB subset. 
% See the help menu for details. 

result=x*0.999+u;
